simulink model "model"  (R2020a)
settings: Solver=VariableStepAuto  StartTime=0.0  StopTime=10.0  RelTol=1e-3
settings Model: Creator=igorbeduin  LastModifiedBy=igorbeduin

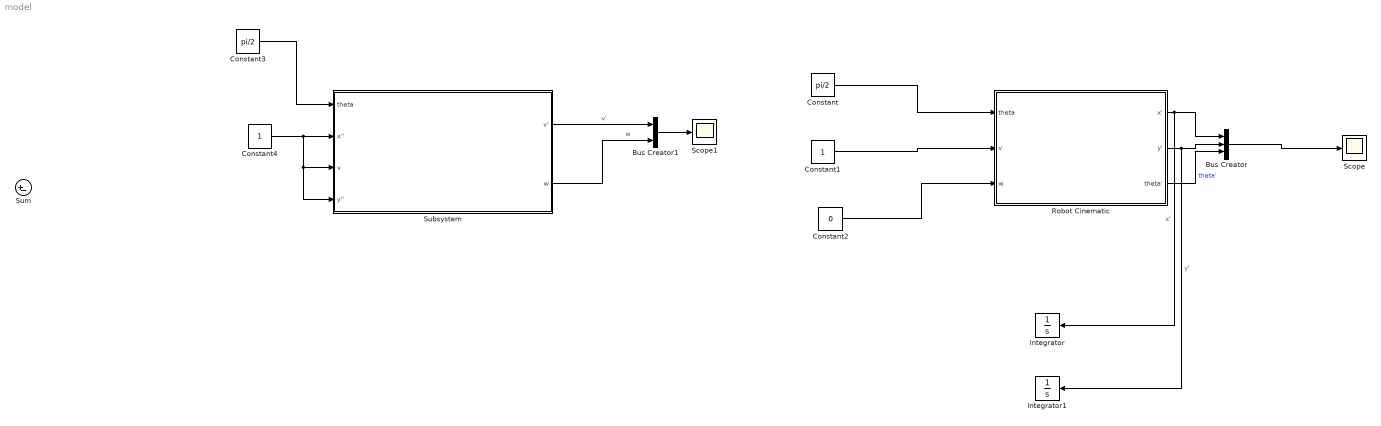
== system model ==
  Bus Creator : BusCreator  Inputs=3
  Bus Creator1 : BusCreator  Inputs=2
  Constant : Constant  Value=pi/2
  Constant1 : Constant
  Constant2 : Constant  Value=0
  Constant3 : Constant  Value=pi/2
  Constant4 : Constant
  Integrator : Integrator
  Integrator1 : Integrator
  Robot Cinematic : Subsystem
  Scope : Scope
  Scope1 : Scope
  Subsystem : Subsystem
  Sum : Sum  Inputs=|+-
  wires:
  Robot Cinematic/1(x') -> Integrator/1, Bus Creator/1  "x'"
  Robot Cinematic/2(y') -> Integrator1/1, Bus Creator/2  "y'"
  Robot Cinematic/3(theta') -> Bus Creator/3  "theta'"
  Bus Creator/1 -> Scope/1
  Constant/1 -> Robot Cinematic/1(theta)
  Constant2/1 -> Robot Cinematic/3(w)
  Constant1/1 -> Robot Cinematic/2(v)
  Constant3/1 -> Subsystem/1(theta)
  Constant4/1 -> Subsystem/2(x''), Subsystem/4(y''), Subsystem/3(v)
  Subsystem/1(v') -> Bus Creator1/1  "v'"
  Subsystem/2(w) -> Bus Creator1/2  "w"
  Bus Creator1/1 -> Scope1/1

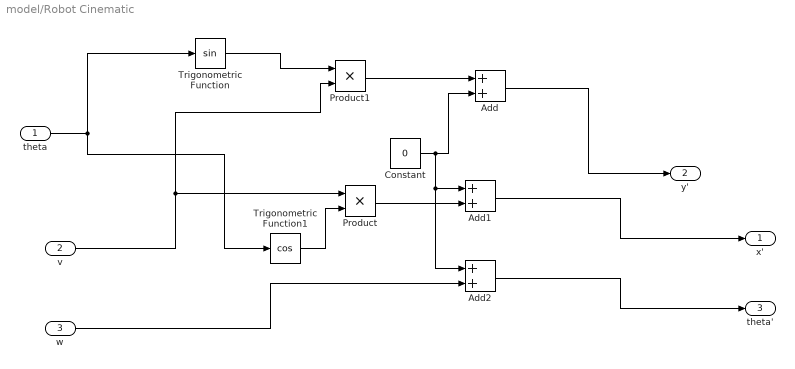
== system model/Robot Cinematic ==
  theta : Inport
  v : Inport  Port=2
  w : Inport  Port=3
  Add : Sum
  Add1 : Sum
  Add2 : Sum
  Constant : Constant  Value=0
  Product : Product
  Product1 : Product
  Trigonometric Function : Trigonometry
  Trigonometric Function1 : Trigonometry  Operator=cos
  x' : Outport
  y' : Outport  Port=2
  theta' : Outport  Port=3
  wires:
  theta/1 -> Trigonometric Function1/1, Trigonometric Function/1
  Trigonometric Function/1 -> Product1/1
  v/1 -> Product1/2, Product/1
  Trigonometric Function1/1 -> Product/2
  Product1/1 -> Add/1
  Constant/1 -> Add2/1, Add1/1, Add/2
  Product/1 -> Add1/2
  Add1/1 -> x'/1
  w/1 -> Add2/2
  Add2/1 -> theta'/1
  Add/1 -> y'/1

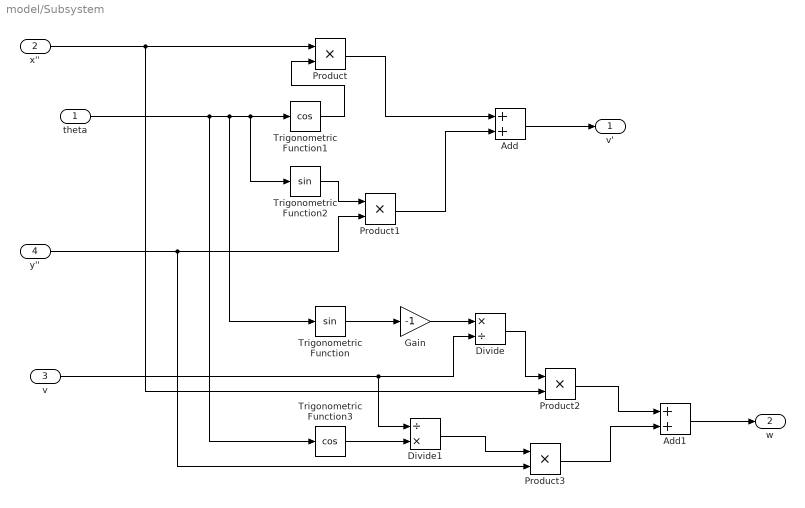
== system model/Subsystem ==
  theta : Inport
  x'' : Inport  Port=2
  v : Inport  Port=3
  y'' : Inport  Port=4
  Add : Sum
  Add1 : Sum
  Divide : Product  Inputs=*/
  Divide1 : Product  Inputs=/*
  Gain : Gain  Gain=-1
  Product{,1..3} (4 alike) : Product
  Trigonometric Function : Trigonometry
  Trigonometric Function1 : Trigonometry  Operator=cos
  Trigonometric Function2 : Trigonometry
  Trigonometric Function3 : Trigonometry  Operator=cos
  v' : Outport
  w : Outport  Port=2
  wires:
  x''/1 -> Product2/2, Product/1
  theta/1 -> Trigonometric Function/1, Trigonometric Function2/1, Trigonometric Function1/1, Trigonometric Function3/1
  Trigonometric Function1/1 -> Product/2
  Product/1 -> Add/1
  Trigonometric Function2/1 -> Product1/1
  y''/1 -> Product3/2, Product1/2
  Product1/1 -> Add/2
  Add/1 -> v'/1
  Trigonometric Function/1 -> Gain/1
  Gain/1 -> Divide/1
  v/1 -> Divide1/1, Divide/2
  Divide/1 -> Product2/1
  Product2/1 -> Add1/1
  Trigonometric Function3/1 -> Divide1/2
  Divide1/1 -> Product3/1
  Product3/1 -> Add1/2
  Add1/1 -> w/1
